simulink model "diskOnPlane_d_V5"  (R2017b)
settings: Solver=VariableStepAuto  StartTime=0.0  StopTime=6  RelTol=1e-3
undefined symbols (not defined in the file): b_contact, cgap, Fz, g, k_contact, mustat, radius, rRim, rTire, s, sigbuilder_block, vthr, X, xPlaLgt, Y, yPlaLgt, Z, zPlaLgt
libraries: sm_lib x23, nesl_utility x14, fl_lib x6, simulink x3, Multibody_Multiphysics_Lib x2, Parts_Lib x1
settings Model: Creator=rizwan  LastModifiedBy=rizwan
settings ExplorerConfigSet: InternalSimMechanicsExplorerSettings="<ExplorerConfiguration><canonicalview>default</canonicalview><AnimationSetting><BasePlaybackSpeed>1.0</BasePlaybackSpeed><PlaybackSpeedFactor>0.5</PlaybackSpeedFactor></AnimationSetting><TilePanel><TileInfo><Tiles Columns=\"1\" Count=\"1\" Rows=\"1\"><Column Weight=\"1\"/><Row Weight=\"1\"/><Tile Height=\"1\" Width=\"1\" X=\"0\" Y=\"0\"/></Tiles></TileInfo><SceneInfo><SceneViewer><BGColor><R>0.60000002384185791</R><G>0.60000002384185791</G><B>0.60000002384185791</B></BGColor><Camera><DoPerspective>off</DoPerspective><Position><X>5.79472373405807684</X><Y>-5.79472391891225325</Y><Z>5.92560694927763798</Z></Position><Center><X>-0.0436274449830504965</X><Y>0.0436272601288755502</Y><Z>0.0872557702365091004</Z></Center><Up><X>-0.408248290463863073</X><Y>0.408248290463863073</Y><Z>0.816496580927726145</Z></Up><ViewLimDist>1</ViewLimDist><YLim>5.77777386756221212</YLim><XLim>8.19359982490539451</XLim></Camera></SceneViewer></SceneInfo></TilePanel><MechEditorPanel><Cameras/><GfxPanelCameraMap/><VideoCreator><PlaybackSpeedRatio>1.0</PlaybackSpeedRatio><FrameRate>30</FrameRate><VideoFormat>Motion JPEG AVI</VideoFormat><FrameSize>auto</FrameSize></VideoCreator></MechEditorPanel></ExplorerConfiguration>"

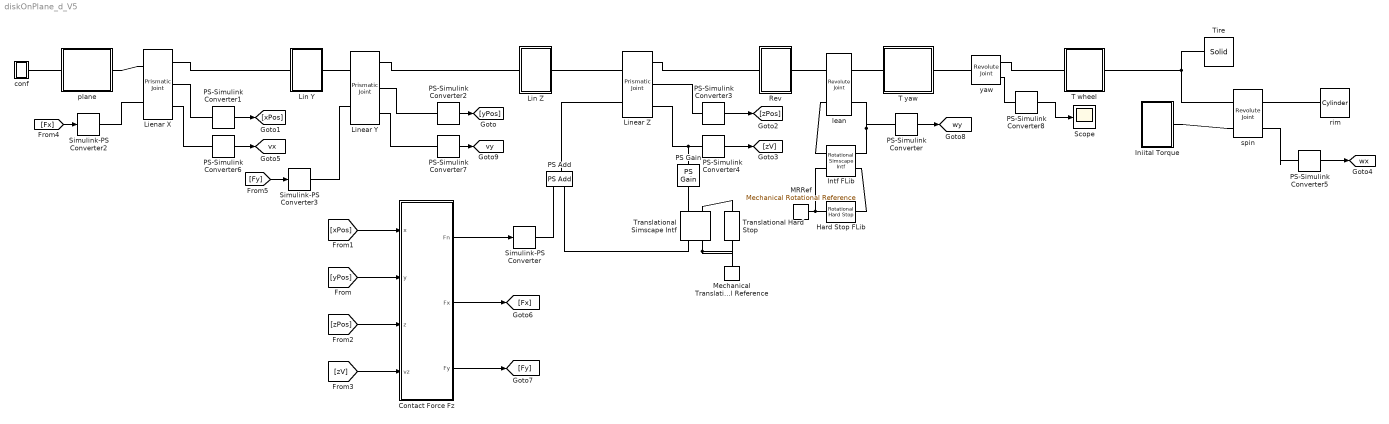
== system diskOnPlane_d_V5 ==
  Contact Force Fz : Subsystem
  Hard Stop FLib : fl_lib/Mechanical/Rotational Elements/Rotational Hard Stop  upper_bnd=70 deg  lower_bnd=-70 deg  stiff_up=1e4 m*N/deg  stiff_low=1e4 m*N/deg  D_up=1e3 m*s*N/deg  D_low=1e3 m*s*N/deg  model=3  transition=0.001 rad  w_specify=off  w_priority=High  w=0 rad/s  w_nominal_specify=off  w_nominal_unit=rad/s  w_nominal_value=1  t_specify=off  t_priority=High  t=0 N*m  t_nominal_specify=off  t_nominal_unit=N*m  t_nominal_value=1  phi_specify=on  phi_priority=High  phi=0 deg  phi_nominal_specify=off  phi_nominal_unit=rad  phi_nominal_value=1
      settings: SourceProductName=Simscape  SourceProductBaseCode=SS
  Iniital Torque : Subsystem
  Intf FLib : Multibody_Multiphysics_Lib/Interfaces/Rotational Simscape Intf  Tag=PublishSubsystem
      settings: SourceProductName=Simscape Multibody Multiphysics Library
  Lienar X : sm_lib/Joints/Prismatic Joint  SenseConstraintForce=off  SenseConstraintForceX=off  SenseConstraintForceY=off  SenseConstraintForceZ=off  SenseConstraintTorque=off  SenseConstraintTorqueX=off  SenseConstraintTorqueY=off  SenseConstraintTorqueZ=off  SenseTotalForce=off  SenseTotalForceX=off  SenseTotalForceY=off  SenseTotalForceZ=off  SenseTotalTorque=off  SenseTotalTorqueX=off  SenseTotalTorqueY=off  SenseTotalTorqueZ=off  CompositeWrenchDir=FollowerOnBase  CompositeWrenchFrame=BaseFrame  EquilibriumPosition=0  EquilibriumPositionUnits=m  SpringStiffness=0  SpringStiffnessUnits=N/m  DampingCoefficient=0  DampingCoefficientUnits=N/(m/s)  TorqueActuationMode=InputTorque  MotionActuationMode=ComputedMotion  SensePosition=on  SenseVelocity=on  SenseAcceleration=off  SenseTorqueForce=off  PositionTargetSpecify=on  PositionTargetPriority=High  PositionTargetValue=sPosX  PositionTargetValueUnits=m  VelocityTargetSpecify=off  VelocityTargetPriority=High  VelocityTargetValue=0  VelocityTargetValueUnits=m/s
  Lin Y : Subsystem
  Lin Z : Subsystem
  Linear Y : sm_lib/Joints/Prismatic Joint  SenseConstraintForce=off  SenseConstraintForceX=off  SenseConstraintForceY=off  SenseConstraintForceZ=off  SenseConstraintTorque=off  SenseConstraintTorqueX=off  SenseConstraintTorqueY=off  SenseConstraintTorqueZ=off  SenseTotalForce=off  SenseTotalForceX=off  SenseTotalForceY=off  SenseTotalForceZ=off  SenseTotalTorque=off  SenseTotalTorqueX=off  SenseTotalTorqueY=off  SenseTotalTorqueZ=off  CompositeWrenchDir=FollowerOnBase  CompositeWrenchFrame=BaseFrame  EquilibriumPosition=0  EquilibriumPositionUnits=m  SpringStiffness=0  SpringStiffnessUnits=N/m  DampingCoefficient=0  DampingCoefficientUnits=N/(m/s)  TorqueActuationMode=InputTorque  MotionActuationMode=ComputedMotion  SensePosition=on  SenseVelocity=on  SenseAcceleration=off  SenseTorqueForce=off  PositionTargetSpecify=off  PositionTargetPriority=High  PositionTargetValue=0  PositionTargetValueUnits=m  VelocityTargetSpecify=off  VelocityTargetPriority=High  VelocityTargetValue=0  VelocityTargetValueUnits=m/s
  Linear Z : sm_lib/Joints/Prismatic Joint  SenseConstraintForce=off  SenseConstraintForceX=off  SenseConstraintForceY=off  SenseConstraintForceZ=off  SenseConstraintTorque=off  SenseConstraintTorqueX=off  SenseConstraintTorqueY=off  SenseConstraintTorqueZ=off  SenseTotalForce=off  SenseTotalForceX=off  SenseTotalForceY=off  SenseTotalForceZ=off  SenseTotalTorque=off  SenseTotalTorqueX=off  SenseTotalTorqueY=off  SenseTotalTorqueZ=off  CompositeWrenchDir=FollowerOnBase  CompositeWrenchFrame=BaseFrame  EquilibriumPosition=0  EquilibriumPositionUnits=m  SpringStiffness=0  SpringStiffnessUnits=N/m  DampingCoefficient=0  DampingCoefficientUnits=N/(m/s)  TorqueActuationMode=InputTorque  MotionActuationMode=ComputedMotion  SensePosition=on  SenseVelocity=on  SenseAcceleration=off  SenseTorqueForce=off  PositionTargetSpecify=off  PositionTargetPriority=High  PositionTargetValue=0  PositionTargetValueUnits=m  VelocityTargetSpecify=off  VelocityTargetPriority=High  VelocityTargetValue=0  VelocityTargetValueUnits=m/s
  MRRef : fl_lib/Mechanical/Rotational Elements/Mechanical Rotational Reference
  Mechanical Translational Reference : fl_lib/Mechanical/Translational Elements/Mechanical Translational Reference
  PS Add : fl_lib/Physical Signals/Functions/PS Add
  PS Gain : fl_lib/Physical Signals/Functions/PS Gain  gain=1
  PS-Simulink Converter{,1..7} (8 alike) : nesl_utility/PS-Simulink Converter  PhysicalDomain=network_engine_domain  SubClassName=ps_output  LeftPortType=input  RightPortType=output  PseudoPeriodic=off  Frequencies=[]  Unit=1  AffineConversion=off
  PS-Simulink Converter8 : nesl_utility/PS-Simulink Converter  PhysicalDomain=network_engine_domain  SubClassName=ps_output  LeftPortType=input  RightPortType=output  PseudoPeriodic=off  Frequencies=[]  Unit=deg  AffineConversion=off
  Rev : Subsystem
  Scope : Scope
  Simulink-PS Converter : nesl_utility/Simulink-PS Converter  PhysicalDomain=network_engine_domain  SubClassName=ps_input  LeftPortType=input  RightPortType=output  PseudoPeriodic=off  Frequencies=[]  NoiseDistribution=none  NoiseParameters=[]  Unit=1  AffineConversion=off  FilteringAndDerivatives=provide  SimscapeFilterOrder=1  InputFilterTimeConstant=0.001  UdotUserProvided=0
  Simulink-PS Converter2 : nesl_utility/Simulink-PS Converter  PhysicalDomain=network_engine_domain  SubClassName=ps_input  LeftPortType=input  RightPortType=output  PseudoPeriodic=off  Frequencies=[]  NoiseDistribution=none  NoiseParameters=[]  Unit=1  AffineConversion=off  FilteringAndDerivatives=provide  SimscapeFilterOrder=1  InputFilterTimeConstant=0.001  UdotUserProvided=0
  Simulink-PS Converter3 : nesl_utility/Simulink-PS Converter  PhysicalDomain=network_engine_domain  SubClassName=ps_input  LeftPortType=input  RightPortType=output  PseudoPeriodic=off  Frequencies=[]  NoiseDistribution=none  NoiseParameters=[]  Unit=1  AffineConversion=off  FilteringAndDerivatives=provide  SimscapeFilterOrder=1  InputFilterTimeConstant=0.001  UdotUserProvided=0
  T wheel : Subsystem
  T yaw : Subsystem
  Tire : sm_lib/Body Elements/Solid  InertiaType=CalculateFromGeometry  Mass=1  MassUnits=kg  CenterOfMass=[0 0 0]  CenterOfMassUnits=m  MomentsOfInertia=[1 1 1]  MomentsOfInertiaUnits=kg*m^2  ProductsOfInertia=[1 1 1]  ProductsOfInertiaUnits=kg*m^2  DensityBased=on  Density=rhoTire  DensityUnits=kg/m^3  DoExposeReferenceFrame=on  SerializedFrames=<Frames/>  GraphicType=FromGeometry  MarkerShape=Sphere  MarkerSize=10  GraphicVisPropType=SimpleVisualProperties  GraphicDiffuseColor=[1.0 0.2 0.2]  GraphicSpecularColor=[0.5 0.5 0.5 1.0]  GraphicAmbientColor=[0.15 0.15 0.15 1.0]  GraphicEmissiveColor=[0.0 0.0 0.0 1.0]  GraphicShininess=75  GraphicOpacity=0.3  GeometryShape=GeneralSolidOfRevolution  RectangleSize=[1 1]  RectangleSizeUnits=m  BrickDimensions=[1 1 1]  BrickDimensionUnits=m  CylinderRadius=1  CylinderRadiusUnits=m  CylinderLength=1  CylinderLengthUnits=m  SphereRadius=1  SphereRadiusUnits=m  EllipsoidRadii=[1 1 1]  EllipsoidRadiiUnits=m  ExtrusionCrossSection=[1 1; -1 1; -1 -1; 1 -1]  ExtrusionCrossSectionUnits=m  ExtrusionLength=1  ExtrusionLengthUnits=m  PolygonNumSides=3  PolygonOuterRadius=1  PolygonOuterRadiusUnits=m  ExtGeomFileType=STEP  ExtGeomFileUnits=m  RevolutionCrossSection=aTire  RevolutionCrossSectionUnits=m  RevolutionExtent=Full  RevolutionAngle=180  RevolutionAngleUnits=deg
  Translational Simscape Intf : Multibody_Multiphysics_Lib/Interfaces/Translational Simscape Intf
  Translational Hard Stop : fl_lib/Mechanical/Translational Elements/Translational Hard Stop  upper_bnd=+inf m  lower_bnd=-inf cm  stiff_up=1e6 N/m  stiff_low=1e6 N/m  D_up=150 N/(m/s)  D_low=150 N/(m/s)  model=3  transition=0.1 mm  v_specify=off  v_priority=None  v=0 m/s  v_nominal_specify=off  v_nominal_unit=m/s  v_nominal_value=1  f_specify=off  f_priority=None  f=0 N  f_nominal_specify=off  f_nominal_unit=N  f_nominal_value=1  x_specify=off  x_priority=High  x=0 m  x_nominal_specify=off  x_nominal_unit=m  x_nominal_value=1
  conf : Subsystem
  lean : sm_lib/Joints/Revolute Joint  SenseConstraintForce=off  SenseConstraintForceX=off  SenseConstraintForceY=off  SenseConstraintForceZ=off  SenseConstraintTorque=off  SenseConstraintTorqueX=off  SenseConstraintTorqueY=off  SenseConstraintTorqueZ=off  SenseTotalForce=off  SenseTotalForceX=off  SenseTotalForceY=off  SenseTotalForceZ=off  SenseTotalTorque=off  SenseTotalTorqueX=off  SenseTotalTorqueY=off  SenseTotalTorqueZ=off  CompositeWrenchDir=FollowerOnBase  CompositeWrenchFrame=BaseFrame  EquilibriumPosition=0  EquilibriumPositionUnits=deg  SpringStiffness=0  SpringStiffnessUnits=N*m/deg  DampingCoefficient=0  DampingCoefficientUnits=N*m/(deg/s)  TorqueActuationMode=InputTorque  MotionActuationMode=ComputedMotion  SensePosition=off  SenseVelocity=on  SenseAcceleration=off  SenseTorqueForce=off  PositionTargetSpecify=on  PositionTargetPriority=High  PositionTargetValue=dAngle  PositionTargetValueUnits=deg  VelocityTargetSpecify=off  VelocityTargetPriority=High  VelocityTargetValue=0  VelocityTargetValueUnits=deg/s
  plane : Subsystem
  rim : Parts_Lib/Cylinder  Tag=CustomStyle  cyl_radius=rRim  cyl_length=lRim  cyl_density=rhoDisk  cyl_color=blue  cyl_opacity=1  cyl_color_custom="[0.7920    0.9900    0.9900]"  mark_radius=[0.75 0.5]  mark_len_factor=1.01  mark_angle=60  mark_color=purple  mark_opacity=1
  spin : sm_lib/Joints/Revolute Joint  SenseConstraintForce=off  SenseConstraintForceX=off  SenseConstraintForceY=off  SenseConstraintForceZ=off  SenseConstraintTorque=off  SenseConstraintTorqueX=off  SenseConstraintTorqueY=off  SenseConstraintTorqueZ=off  SenseTotalForce=off  SenseTotalForceX=off  SenseTotalForceY=off  SenseTotalForceZ=off  SenseTotalTorque=off  SenseTotalTorqueX=off  SenseTotalTorqueY=off  SenseTotalTorqueZ=off  CompositeWrenchDir=FollowerOnBase  CompositeWrenchFrame=BaseFrame  EquilibriumPosition=0  EquilibriumPositionUnits=deg  SpringStiffness=0  SpringStiffnessUnits=N*m/deg  DampingCoefficient=0  DampingCoefficientUnits=N*m/(deg/s)  TorqueActuationMode=InputTorque  MotionActuationMode=ComputedMotion  SensePosition=off  SenseVelocity=on  SenseAcceleration=off  SenseTorqueForce=off  PositionTargetSpecify=off  PositionTargetPriority=High  PositionTargetValue=0  PositionTargetValueUnits=deg  VelocityTargetSpecify=off  VelocityTargetPriority=High  VelocityTargetValue=0  VelocityTargetValueUnits=deg/s
  yaw : sm_lib/Joints/Revolute Joint  SenseConstraintForce=off  SenseConstraintForceX=off  SenseConstraintForceY=off  SenseConstraintForceZ=off  SenseConstraintTorque=off  SenseConstraintTorqueX=off  SenseConstraintTorqueY=off  SenseConstraintTorqueZ=off  SenseTotalForce=off  SenseTotalForceX=off  SenseTotalForceY=off  SenseTotalForceZ=off  SenseTotalTorque=off  SenseTotalTorqueX=off  SenseTotalTorqueY=off  SenseTotalTorqueZ=off  CompositeWrenchDir=FollowerOnBase  CompositeWrenchFrame=BaseFrame  EquilibriumPosition=0  EquilibriumPositionUnits=deg  SpringStiffness=0  SpringStiffnessUnits=N*m/deg  DampingCoefficient=0  DampingCoefficientUnits=N*m/(deg/s)  TorqueActuationMode=NoTorque  MotionActuationMode=ComputedMotion  SensePosition=on  SenseVelocity=off  SenseAcceleration=off  SenseTorqueForce=off  PositionTargetSpecify=off  PositionTargetPriority=High  PositionTargetValue=0  PositionTargetValueUnits=deg  VelocityTargetSpecify=off  VelocityTargetPriority=High  VelocityTargetValue=0  VelocityTargetValueUnits=deg/s
  tag scope: vx=global, vy=global, wx=global, wy=global
  wires:
  PS-Simulink Converter5/1 -> [wx]
  PS-Simulink Converter/1 -> [wy]
  [Fx] -> Simulink-PS Converter2/1
  PS-Simulink Converter1/1 -> [xPos]
  PS-Simulink Converter6/1 -> [vx]
  [Fy] -> Simulink-PS Converter3/1
  PS-Simulink Converter2/1 -> [yPos]
  PS-Simulink Converter7/1 -> [vy]
  PS-Simulink Converter4/1 -> [zV]
  PS-Simulink Converter3/1 -> [zPos]
  Contact Force Fz/1(Fn) -> Simulink-PS Converter/1
  [xPos] -> Contact Force Fz/1(x)
  [yPos] -> Contact Force Fz/2(y)
  Contact Force Fz/3(Fy) -> [Fy]
  [zV] -> Contact Force Fz/4(vz)
  [zPos] -> Contact Force Fz/3(z)
  Contact Force Fz/2(Fx) -> [Fx]
  PS-Simulink Converter8/1 -> Scope/1
  connections:
  Tire/RConn1 -- T wheel/RConn1 -- spin/LConn1
  plane/LConn1 -- conf/RConn1
  plane/RConn1 -- Lienar X/LConn1
  Lienar X/RConn1 -- Lin Y/LConn1
  Linear Y/LConn1 -- Lin Y/RConn1
  Lin Z/LConn1 -- Linear Y/RConn1
  Linear Z/LConn1 -- Lin Z/RConn1
  Rev/LConn1 -- Linear Z/RConn1
  lean/LConn1 -- Rev/RConn1
  T yaw/LConn1 -- lean/RConn1
  T yaw/RConn1 -- yaw/LConn1
  spin/RConn1 -- rim/LConn1
  spin/RConn2 -- PS-Simulink Converter5/LConn1
  yaw/RConn1 -- T wheel/LConn1
  lean/RConn2 -- PS-Simulink Converter/LConn1 -- Intf FLib/RConn1
  Intf FLib/LConn1 -- lean/LConn2
  Hard Stop FLib/LConn1 -- Intf FLib/RConn2
  Hard Stop FLib/RConn1 -- MRRef/LConn1 -- Intf FLib/LConn2
  Simulink-PS Converter2/RConn1 -- Lienar X/LConn2
  Lienar X/RConn2 -- PS-Simulink Converter1/LConn1
  Lienar X/RConn3 -- PS-Simulink Converter6/LConn1
  Iniital Torque/RConn1 -- spin/LConn2
  Linear Y/LConn2 -- Simulink-PS Converter3/RConn1
  Linear Y/RConn2 -- PS-Simulink Converter2/LConn1
  PS-Simulink Converter7/LConn1 -- Linear Y/RConn3
  Linear Z/RConn2 -- PS-Simulink Converter3/LConn1
  Linear Z/RConn3 -- PS Gain/LConn1 -- PS-Simulink Converter4/LConn1
  Translational Simscape Intf/LConn2 -- Translational Hard Stop/RConn1 -- Mechanical Translational Reference/LConn1
  PS Gain/RConn1 -- Translational Simscape Intf/RConn1
  Translational Simscape Intf/LConn1 -- PS Add/LConn1
  Translational Hard Stop/LConn1 -- Translational Simscape Intf/RConn2
  Simulink-PS Converter/RConn1 -- PS Add/LConn2
  PS Add/RConn1 -- Linear Z/LConn2
  PS-Simulink Converter8/LConn1 -- yaw/RConn2

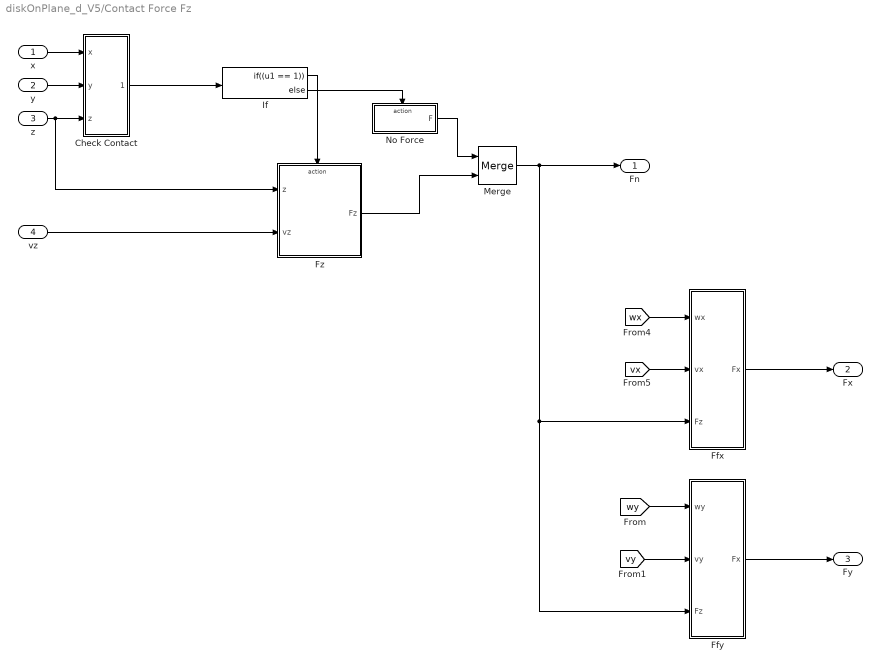
== system diskOnPlane_d_V5/Contact Force Fz ==
  x : Inport
  y : Inport  Port=2
  z : Inport  Port=3
  vz : Inport  Port=4
  Check Contact : Subsystem
  Ffx : Subsystem
  Ffy : Subsystem
  Fz : Subsystem
  If : If  IfExpression=(u1 == 1)
  Merge : Merge  InitialOutput=0  InputPortOffsets=0
  No Force : Subsystem  AncestorBlock=Contact_Forces_Lib/2D/Circle to Finite Line Force/No Force
  Fn : Outport
  Fx : Outport  Port=2
  Fy : Outport  Port=3
  wires:
  Fz/1(Fz) -> Merge/2
  If/1 -> Fz/Action
  Check Contact/1(Enable) -> If/1
  No Force/1(F) -> Merge/1
  Merge/1 -> Ffy/3(Fz), Ffx/3(Fz), Fn/1
  x/1 -> Check Contact/1(x)
  If/2 -> No Force/Action
  y/1 -> Check Contact/2(y)
  z/1 -> Fz/1(z), Check Contact/3(z)
  vz/1 -> Fz/2(vz)
  [vx] -> Ffx/2(vx)
  [wx] -> Ffx/1(wx)
  Ffx/1(Fx) -> Fx/1
  [wy] -> Ffy/1(wy)
  [vy] -> Ffy/2(vy)
  Ffy/1(Fx) -> Fy/1

== system diskOnPlane_d_V5/Iniital Torque ==
  Gain : Gain  Gain=1/2.5
  Signal Builder : Subsystem  Tag=STV Subsys  LoadFcn=sigbuilder_block('load');  StartFcn=sigbuilder_block('start');  StopFcn=sigbuilder_block('stop');  ClipboardFcn=sigbuilder_block('clipboard');  mask(Sigbuilder block){tuvar=[0:10]}
      mask help: Simulink:masks:SigbuilderBlock_MD
      mask init:
      | if ~strcmp(get_param(bdroot(gcbh),'SimulationStatus'),'stopped') tuvar = sigbuilder_block('maskInit'); end
      settings: CopyFcn=sigbuilder_block('copy');  DeleteFcn=sigbuilder_block('delete');  ModelCloseFcn=sigbuilder_block('modelClose');  PreSaveFcn=sigbuilder_block('preSave');  PauseFcn=sigbuilder_block('pause');  ContinueFcn=sigbuilder_block('continue');  NameChangeFcn=sigbuilder_block('namechange');  OpenFcn=sigbuilder_block('open',[48.75 0 975.75 495.75 ]);  CloseFcn=sigbuilder_block('close');
      mask Display: plot(0, 0, 100, 100,[2, 2, 32, 32, 2], [68, 8, 8, 68, 68],[32, 2], [38, 38], [32, 19, 2],[53, 60, 44], [32, 17, 17, 2],[16, 16, 31, 31]);txt = getActiveGroup(gcbh);text(2, 100, txt,'verticalAlignment', 'top');
  Simulink-PS Converter1 : nesl_utility/Simulink-PS Converter  PhysicalDomain=network_engine_domain  SubClassName=ps_input  LeftPortType=input  RightPortType=output  PseudoPeriodic=off  Frequencies=[]  NoiseDistribution=none  NoiseParameters=[]  Unit=N*m  AffineConversion=off  FilteringAndDerivatives=filter  SimscapeFilterOrder=2  InputFilterTimeConstant=0.1  UdotUserProvided=0
  wheel : PMIOPort  Port=1  Side=Right
  wires:
  Gain/1 -> Simulink-PS Converter1/1
  Signal Builder/1(Signal 1) -> Gain/1
  connections:
  Simulink-PS Converter1/RConn1 -- wheel/RConn1

== system diskOnPlane_d_V5/Lin Y ==
  Rev for Linear X : sm_lib/Frames and Transforms/Rigid Transform  TranslationMethod=None  TranslationStandardOffset=0  TranslationLengthUnit=m  TranslationStandardAxis=+Z  TranslationCartesianOffset=[0 0 0]  TranslationROffset=0  TranslationROffsetUnits=m  TranslationZOffset=0  TranslationZOffsetUnits=m  TranslationThetaOffset=0  TranslationThetaOffsetUnits=deg  RotationMethod=StandardAxis  RotationAngleUnits=deg  RotationStandardAxis=-Y  RotationAngle=90  RotationArbitraryAxis=[0 0 1]  FollAlignAxisA=+X  BaseAlignAxisA=+Y  FollAlignAxisB=+Y  BaseAlignAxisB=+Z  RotationSequenceAxes=FollowerAxes  RotationSequence=XYX  RotationSequenceAngles=[0 0 0]  RotationSequenceAnglesUnits=deg  RotationMatrix=[1 0 0; 0 1 0; 0 0 1]
  Trans for Linear Y : sm_lib/Frames and Transforms/Rigid Transform  TranslationMethod=StandardAxis  TranslationStandardOffset=rTire  TranslationLengthUnit=m  TranslationStandardAxis=-Y  TranslationCartesianOffset=[0 0 0]  TranslationROffset=0  TranslationROffsetUnits=m  TranslationZOffset=0  TranslationZOffsetUnits=m  TranslationThetaOffset=0  TranslationThetaOffsetUnits=deg  RotationMethod=None  RotationAngleUnits=deg  RotationStandardAxis=+Z  RotationAngle=0.0  RotationArbitraryAxis=[0 0 1]  FollAlignAxisA=+X  BaseAlignAxisA=+Y  FollAlignAxisB=+Y  BaseAlignAxisB=+Z  RotationSequenceAxes=FollowerAxes  RotationSequence=XYX  RotationSequenceAngles=[0 0 0]  RotationSequenceAnglesUnits=deg  RotationMatrix=[1 0 0; 0 1 0; 0 0 1]
  B : PMIOPort  Port=1  Side=Left
  F : PMIOPort  Port=2  Side=Right
  connections:
  B/RConn1 -- Rev for Linear X/LConn1
  F/RConn1 -- Trans for Linear Y/RConn1
  Trans for Linear Y/LConn1 -- Rev for Linear X/RConn1

== system diskOnPlane_d_V5/Lin Z ==
  Rev for Linear Y : sm_lib/Frames and Transforms/Rigid Transform  TranslationMethod=StandardAxis  TranslationStandardOffset=rTire  TranslationLengthUnit=m  TranslationStandardAxis=+Y  TranslationCartesianOffset=[0 0 0]  TranslationROffset=0  TranslationROffsetUnits=m  TranslationZOffset=0  TranslationZOffsetUnits=m  TranslationThetaOffset=0  TranslationThetaOffsetUnits=deg  RotationMethod=None  RotationAngleUnits=deg  RotationStandardAxis=+Z  RotationAngle=0.0  RotationArbitraryAxis=[0 0 1]  FollAlignAxisA=+X  BaseAlignAxisA=+Y  FollAlignAxisB=+Y  BaseAlignAxisB=+Z  RotationSequenceAxes=FollowerAxes  RotationSequence=XYX  RotationSequenceAngles=[0 0 0]  RotationSequenceAnglesUnits=deg  RotationMatrix=[1 0 0; 0 1 0; 0 0 1]
  Trans for Lineaer Z : sm_lib/Frames and Transforms/Rigid Transform  TranslationMethod=None  TranslationStandardOffset=0  TranslationLengthUnit=m  TranslationStandardAxis=+Z  TranslationCartesianOffset=[0 0 0]  TranslationROffset=0  TranslationROffsetUnits=m  TranslationZOffset=0  TranslationZOffsetUnits=m  TranslationThetaOffset=0  TranslationThetaOffsetUnits=deg  RotationMethod=StandardAxis  RotationAngleUnits=deg  RotationStandardAxis=-X  RotationAngle=90  RotationArbitraryAxis=[0 0 1]  FollAlignAxisA=+X  BaseAlignAxisA=+Y  FollAlignAxisB=+Y  BaseAlignAxisB=+Z  RotationSequenceAxes=FollowerAxes  RotationSequence=XYX  RotationSequenceAngles=[0 0 0]  RotationSequenceAnglesUnits=deg  RotationMatrix=[1 0 0; 0 1 0; 0 0 1]
  B : PMIOPort  Port=1  Side=Left
  F : PMIOPort  Port=2  Side=Right
  connections:
  Rev for Linear Y/LConn1 -- B/RConn1
  F/RConn1 -- Trans for Lineaer Z/RConn1
  Trans for Lineaer Z/LConn1 -- Rev for Linear Y/RConn1

== system diskOnPlane_d_V5/Rev ==
  Rev for Linear Z : sm_lib/Frames and Transforms/Rigid Transform  TranslationMethod=None  TranslationStandardOffset=0  TranslationLengthUnit=m  TranslationStandardAxis=+Z  TranslationCartesianOffset=[0 0 0]  TranslationROffset=0  TranslationROffsetUnits=m  TranslationZOffset=0  TranslationZOffsetUnits=m  TranslationThetaOffset=0  TranslationThetaOffsetUnits=deg  RotationMethod=StandardAxis  RotationAngleUnits=deg  RotationStandardAxis=+X  RotationAngle=90  RotationArbitraryAxis=[0 0 1]  FollAlignAxisA=+X  BaseAlignAxisA=+Y  FollAlignAxisB=+Y  BaseAlignAxisB=+Z  RotationSequenceAxes=FollowerAxes  RotationSequence=XYX  RotationSequenceAngles=[0 0 0]  RotationSequenceAnglesUnits=deg  RotationMatrix=[1 0 0; 0 1 0; 0 0 1]
  Trans for lean axis : sm_lib/Frames and Transforms/Rigid Transform  TranslationMethod=StandardAxis  TranslationStandardOffset=rTire  TranslationLengthUnit=m  TranslationStandardAxis=-Y  TranslationCartesianOffset=[0 0 0]  TranslationROffset=0  TranslationROffsetUnits=m  TranslationZOffset=0  TranslationZOffsetUnits=m  TranslationThetaOffset=0  TranslationThetaOffsetUnits=deg  RotationMethod=StandardAxis  RotationAngleUnits=deg  RotationStandardAxis=+Y  RotationAngle=90  RotationArbitraryAxis=[0 0 1]  FollAlignAxisA=+X  BaseAlignAxisA=+Y  FollAlignAxisB=+Y  BaseAlignAxisB=+Z  RotationSequenceAxes=FollowerAxes  RotationSequence=XYX  RotationSequenceAngles=[0 0 0]  RotationSequenceAnglesUnits=deg  RotationMatrix=[1 0 0; 0 1 0; 0 0 1]
  B : PMIOPort  Port=1  Side=Left
  F : PMIOPort  Port=2  Side=Right
  connections:
  Trans for lean axis/LConn1 -- Rev for Linear Z/RConn1
  F/RConn1 -- Trans for lean axis/RConn1
  Rev for Linear Z/LConn1 -- B/RConn1

== system diskOnPlane_d_V5/T wheel ==
  RTrans for yaw axis : sm_lib/Frames and Transforms/Rigid Transform  TranslationMethod=StandardAxis  TranslationStandardOffset=rTire  TranslationLengthUnit=m  TranslationStandardAxis=+Y  TranslationCartesianOffset=[0 0 0]  TranslationROffset=0  TranslationROffsetUnits=m  TranslationZOffset=0  TranslationZOffsetUnits=m  TranslationThetaOffset=0  TranslationThetaOffsetUnits=deg  RotationMethod=None  RotationAngleUnits=deg  RotationStandardAxis=+Z  RotationAngle=0.0  RotationArbitraryAxis=[0 0 1]  FollAlignAxisA=+X  BaseAlignAxisA=+Y  FollAlignAxisB=+Y  BaseAlignAxisB=+Z  RotationSequenceAxes=FollowerAxes  RotationSequence=XYX  RotationSequenceAngles=[0 0 0]  RotationSequenceAnglesUnits=deg  RotationMatrix=[1 0 0; 0 1 0; 0 0 1]
  Rot for yaw axis1 : sm_lib/Frames and Transforms/Rigid Transform  TranslationMethod=None  TranslationStandardOffset=0  TranslationLengthUnit=m  TranslationStandardAxis=+Z  TranslationCartesianOffset=[0 0 0]  TranslationROffset=0  TranslationROffsetUnits=m  TranslationZOffset=0  TranslationZOffsetUnits=m  TranslationThetaOffset=0  TranslationThetaOffsetUnits=deg  RotationMethod=StandardAxis  RotationAngleUnits=deg  RotationStandardAxis=+X  RotationAngle=90  RotationArbitraryAxis=[0 0 1]  FollAlignAxisA=+X  BaseAlignAxisA=+Y  FollAlignAxisB=+Y  BaseAlignAxisB=+Z  RotationSequenceAxes=FollowerAxes  RotationSequence=XYX  RotationSequenceAngles=[0 0 0]  RotationSequenceAnglesUnits=deg  RotationMatrix=[1 0 0; 0 1 0; 0 0 1]
  B : PMIOPort  Port=1  Side=Left
  F : PMIOPort  Port=2  Side=Right
  connections:
  B/RConn1 -- Rot for yaw axis1/LConn1
  Rot for yaw axis1/RConn1 -- RTrans for yaw axis/LConn1
  RTrans for yaw axis/RConn1 -- F/RConn1

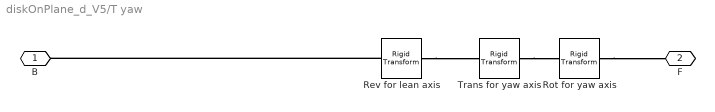
== system diskOnPlane_d_V5/T yaw ==
  Rev for lean axis : sm_lib/Frames and Transforms/Rigid Transform  TranslationMethod=StandardAxis  TranslationStandardOffset=rTire  TranslationLengthUnit=m  TranslationStandardAxis=+Y  TranslationCartesianOffset=[0 0 0]  TranslationROffset=0  TranslationROffsetUnits=m  TranslationZOffset=0  TranslationZOffsetUnits=m  TranslationThetaOffset=0  TranslationThetaOffsetUnits=deg  RotationMethod=StandardAxis  RotationAngleUnits=deg  RotationStandardAxis=-Y  RotationAngle=90  RotationArbitraryAxis=[0 0 1]  FollAlignAxisA=+X  BaseAlignAxisA=+Y  FollAlignAxisB=+Y  BaseAlignAxisB=+Z  RotationSequenceAxes=FollowerAxes  RotationSequence=XYX  RotationSequenceAngles=[0 0 0]  RotationSequenceAnglesUnits=deg  RotationMatrix=[1 0 0; 0 1 0; 0 0 1]
  Rot for yaw axis : sm_lib/Frames and Transforms/Rigid Transform  TranslationMethod=None  TranslationStandardOffset=0  TranslationLengthUnit=m  TranslationStandardAxis=+Z  TranslationCartesianOffset=[0 0 0]  TranslationROffset=0  TranslationROffsetUnits=m  TranslationZOffset=0  TranslationZOffsetUnits=m  TranslationThetaOffset=0  TranslationThetaOffsetUnits=deg  RotationMethod=StandardAxis  RotationAngleUnits=deg  RotationStandardAxis=-X  RotationAngle=90  RotationArbitraryAxis=[0 0 1]  FollAlignAxisA=+X  BaseAlignAxisA=+Y  FollAlignAxisB=+Y  BaseAlignAxisB=+Z  RotationSequenceAxes=FollowerAxes  RotationSequence=XYX  RotationSequenceAngles=[0 0 0]  RotationSequenceAnglesUnits=deg  RotationMatrix=[1 0 0; 0 1 0; 0 0 1]
  Trans for yaw axis : sm_lib/Frames and Transforms/Rigid Transform  TranslationMethod=StandardAxis  TranslationStandardOffset=rTire  TranslationLengthUnit=m  TranslationStandardAxis=-Y  TranslationCartesianOffset=[0 0 0]  TranslationROffset=0  TranslationROffsetUnits=m  TranslationZOffset=0  TranslationZOffsetUnits=m  TranslationThetaOffset=0  TranslationThetaOffsetUnits=deg  RotationMethod=None  RotationAngleUnits=deg  RotationStandardAxis=+Z  RotationAngle=0.0  RotationArbitraryAxis=[0 0 1]  FollAlignAxisA=+X  BaseAlignAxisA=+Y  FollAlignAxisB=+Y  BaseAlignAxisB=+Z  RotationSequenceAxes=FollowerAxes  RotationSequence=XYX  RotationSequenceAngles=[0 0 0]  RotationSequenceAnglesUnits=deg  RotationMatrix=[1 0 0; 0 1 0; 0 0 1]
  B : PMIOPort  Port=1  Side=Left
  F : PMIOPort  Port=2  Side=Right
  connections:
  Trans for yaw axis/RConn1 -- Rot for yaw axis/LConn1
  Rot for yaw axis/RConn1 -- F/RConn1
  Rev for lean axis/LConn1 -- B/RConn1
  Rev for lean axis/RConn1 -- Trans for yaw axis/LConn1

== system diskOnPlane_d_V5/conf ==
  Mechanism Configuration : sm_lib/Utilities/Mechanism Configuration  UniformGravity=Constant  GravityVector=[0 0 -g]  GravityUnits=m/s^2  LinearizationDelta=0.001
  Solver Configuration : nesl_utility/Solver Configuration  PhysicalDomain=network_engine_domain  SubClassName=solver  LeftPortType=input  RightPortType=generic  Accelerate=off  Tones=[]  Harmonics=[]  SimulateNoise=off  Profile=off  UseLocalSampling=off  EnableSwitchedLinearOptims=on  FrequencyDomain=off  UseCCode=off  RelTol=0.001  AbsTol=1e-06  MinStep=1e-09  ToWorkspace=off  RevertToSquareIcSolve=off  NumHomotopyIterations=100  PhasorMode=off  PhasorModeNumHarmonics=1  DoDC=off  ResidualTolerance=1e-9  UseLocalSolver=off  LocalSolverChoice=NE_BACKWARD_EULER_ADVANCER  LocalSolverSampleTime=.001  DoFixedCost=off  MaxNonlinIter=3  MaxModeIter=2  LinearAlgebra=Sparse  DelaysMemoryBudget=1024  AutomaticFiltering=on  FilteringTimeConstant=0.001
  World Frame : sm_lib/Frames and Transforms/World Frame
  c : PMIOPort  Port=1  Side=Right
  connections:
  Mechanism Configuration/RConn1 -- Solver Configuration/RConn1 -- c/RConn1 -- World Frame/RConn1

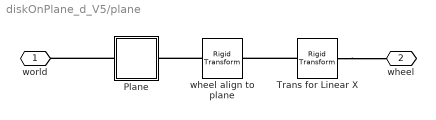
== system diskOnPlane_d_V5/plane ==
  Plane : Subsystem
  Trans for Linear X : sm_lib/Frames and Transforms/Rigid Transform  TranslationMethod=None  TranslationStandardOffset=0  TranslationLengthUnit=m  TranslationStandardAxis=+Z  TranslationCartesianOffset=[0 0 0]  TranslationROffset=0  TranslationROffsetUnits=m  TranslationZOffset=0  TranslationZOffsetUnits=m  TranslationThetaOffset=0  TranslationThetaOffsetUnits=deg  RotationMethod=StandardAxis  RotationAngleUnits=deg  RotationStandardAxis=+Y  RotationAngle=90  RotationArbitraryAxis=[0 0 1]  FollAlignAxisA=+X  BaseAlignAxisA=+Y  FollAlignAxisB=+Y  BaseAlignAxisB=+Z  RotationSequenceAxes=FollowerAxes  RotationSequence=XYX  RotationSequenceAngles=[0 0 0]  RotationSequenceAnglesUnits=deg  RotationMatrix=[1 0 0; 0 1 0; 0 0 1]
  wheel align to plane : sm_lib/Frames and Transforms/Rigid Transform  TranslationMethod=Cartesian  TranslationStandardOffset=radius+zPlaLgt/2  TranslationLengthUnit=m  TranslationStandardAxis=+Z  TranslationCartesianOffset=[0 0 rRim+s+zPlaLgt/2]  TranslationROffset=0  TranslationROffsetUnits=m  TranslationZOffset=0  TranslationZOffsetUnits=m  TranslationThetaOffset=0  TranslationThetaOffsetUnits=deg  RotationMethod=StandardAxis  RotationAngleUnits=deg  RotationStandardAxis=+X  RotationAngle=90  RotationArbitraryAxis=[0 0 1]  FollAlignAxisA=+X  BaseAlignAxisA=+Y  FollAlignAxisB=+Y  BaseAlignAxisB=+Z  RotationSequenceAxes=FollowerAxes  RotationSequence=XYX  RotationSequenceAngles=[0 0 0]  RotationSequenceAnglesUnits=deg  RotationMatrix=[1 0 0; 0 1 0; 0 0 1]
  world : PMIOPort  Port=1  Side=Left
  wheel : PMIOPort  Port=2  Side=Right
  connections:
  Plane/LConn1 -- world/RConn1
  wheel align to plane/LConn1 -- Plane/RConn1
  Trans for Linear X/LConn1 -- wheel align to plane/RConn1
  Trans for Linear X/RConn1 -- wheel/RConn1

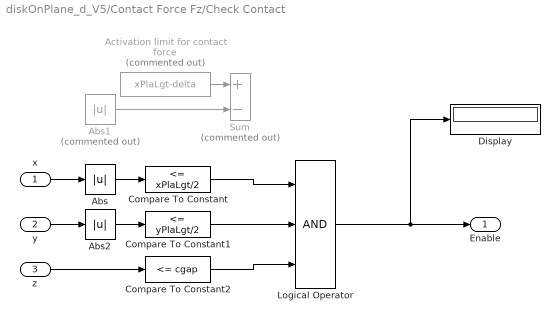
== system diskOnPlane_d_V5/Contact Force Fz/Check Contact ==
  x : Inport
  y : Inport  Port=2
  z : Inport  Port=3
  Abs : Abs
  Abs1 : Abs  Commented=on  ZeroCross=off
  Abs2 : Abs
  Activation limit for contact force : Constant  Commented=on  Value=xPlaLgt-delta
  Compare To Constant : simulink/Logic and Bit Operations/Compare To Constant  relop=<=  const=xPlaLgt/2  OutDataTypeStr=boolean
  Compare To Constant1 : simulink/Logic and Bit Operations/Compare To Constant  relop=<=  const=yPlaLgt/2  OutDataTypeStr=boolean
  Compare To Constant2 : simulink/Logic and Bit Operations/Compare To Constant  relop=<=  const=cgap  OutDataTypeStr=boolean
  Display : Display
  Logical Operator : Logic  Inputs=3  AllPortsSameDT=off  OutDataTypeStr=boolean
  Sum : Sum  Commented=on  Inputs=+-
  Enable : Outport
  wires:
  Activation limit for contact force/1 -> Sum/1
  Abs1/1 -> Sum/2
  x/1 -> Abs/1
  y/1 -> Abs2/1
  Abs/1 -> Compare To Constant/1
  Abs2/1 -> Compare To Constant1/1
  z/1 -> Compare To Constant2/1
  Compare To Constant1/1 -> Logical Operator/2
  Compare To Constant/1 -> Logical Operator/1
  Compare To Constant2/1 -> Logical Operator/3
  Logical Operator/1 -> Display/1, Enable/1

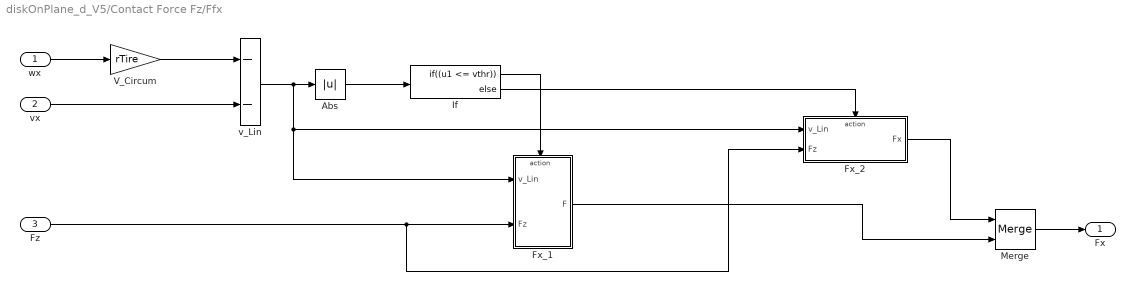
== system diskOnPlane_d_V5/Contact Force Fz/Ffx ==
  wx : Inport
  vx : Inport  Port=2
  Fz : Inport  Port=3
  Abs : Abs
  Fx_1 : Subsystem  AncestorBlock=Contact_Forces_Lib/2D/Circle to Finite Line Force/No Force
  Fx_2 : Subsystem
  If : If  IfExpression=(u1 <= vthr)
  Merge : Merge
  V_Circum : Gain  Gain=rTire
  v_Lin : Sum  Inputs=--
  Fx : Outport
  wires:
  wx/1 -> V_Circum/1
  V_Circum/1 -> v_Lin/1
  vx/1 -> v_Lin/2
  v_Lin/1 -> Fx_2/1(v_Lin), Fx_1/1(v_Lin), Abs/1
  Abs/1 -> If/1
  If/1 -> Fx_1/Action
  Fz/1 -> Fx_2/2(Fz), Fx_1/2(Fz)
  If/2 -> Fx_2/Action
  Merge/1 -> Fx/1
  Fx_1/1(F) -> Merge/2
  Fx_2/1(Fx) -> Merge/1

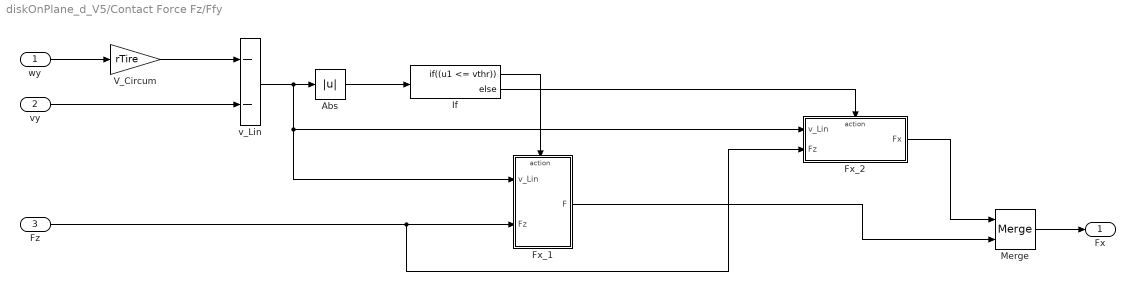
== system diskOnPlane_d_V5/Contact Force Fz/Ffy ==
  wy : Inport
  vy : Inport  Port=2
  Fz : Inport  Port=3
  Abs : Abs
  Fx_1 : Subsystem  AncestorBlock=Contact_Forces_Lib/2D/Circle to Finite Line Force/No Force
  Fx_2 : Subsystem
  If : If  IfExpression=(u1 <= vthr)
  Merge : Merge
  V_Circum : Gain  Gain=rTire
  v_Lin : Sum  Inputs=--
  Fx : Outport
  wires:
  Fx_2/1(Fx) -> Merge/1
  Fx_1/1(F) -> Merge/2
  Merge/1 -> Fx/1
  If/2 -> Fx_2/Action
  Fz/1 -> Fx_1/2(Fz), Fx_2/2(Fz)
  If/1 -> Fx_1/Action
  Abs/1 -> If/1
  v_Lin/1 -> Abs/1, Fx_1/1(v_Lin), Fx_2/1(v_Lin)
  vy/1 -> v_Lin/2
  V_Circum/1 -> v_Lin/1
  wy/1 -> V_Circum/1

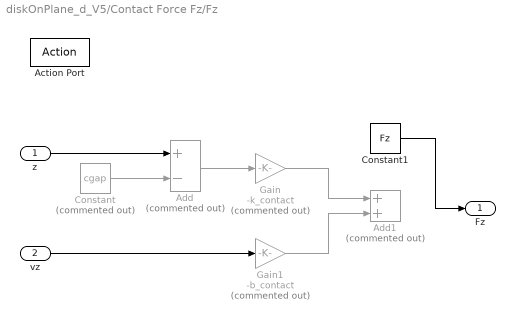
== system diskOnPlane_d_V5/Contact Force Fz/Fz ==
  z : Inport
  vz : Inport  Port=2
  Action Port : ActionPort  ActionType=then
  Add : Sum  Commented=on  Inputs=+-
  Add1 : Sum  Commented=on
  Constant : Constant  Commented=on  Value=cgap
  Constant1 : Constant  Value=Fz
  Gain : Gain  Commented=on  Gain=-k_contact
  Gain1 : Gain  Commented=on  Gain=-b_contact
  Fz : Outport
  wires:
  z/1 -> Add/1
  Constant/1 -> Add/2
  Add/1 -> Gain/1
  vz/1 -> Gain1/1
  Gain/1 -> Add1/1
  Gain1/1 -> Add1/2
  Constant1/1 -> Fz/1

== system diskOnPlane_d_V5/Contact Force Fz/No Force ==
  Action Port : ActionPort  ActionType=else
  Zeros : Constant  Value=0  SampleTime=0
  F : Outport  InitialOutput=0
  wires:
  Zeros/1 -> F/1

== system diskOnPlane_d_V5/Iniital Torque/Signal Builder ==
  Demux : Demux  Tag=STV Demux  Outputs=1
  FromWs : FromWorkspace  Tag=STV FromWs  VariableName=tuvar  SampleTime=0
      SigBuilderData=|
      | common.afterFinalStr = 'Extrapolate'
      | common.sampleTime = 0
      | dataSet.timeRange = [0 10]
      | dataSet.name = 'Group 1'
      | sbobj.Groups.Name = 'Group 1'
      | sbobj.Groups.Signals.Name = 'Signal 1'
      | sbobj.Groups.Signals.XData = [0 1 1 10]
      | sbobj.Groups.Signals.YData = [-500 -500 0 0]
  Signal 1 : Outport  Tag=STV Outport
  wires:
  Demux/1 -> Signal 1/1
  FromWs/1 -> Demux/1

== system diskOnPlane_d_V5/plane/Plane ==
  Plane : sm_lib/Body Elements/Solid  InertiaType=CalculateFromGeometry  Mass=1  MassUnits=kg  CenterOfMass=[0 0 0]  CenterOfMassUnits=m  MomentsOfInertia=[1 1 1]  MomentsOfInertiaUnits=kg*m^2  ProductsOfInertia=[0 0 0]  ProductsOfInertiaUnits=kg*m^2  DensityBased=on  Density=1000  DensityUnits=kg/(m^3)  DoExposeReferenceFrame=on  SerializedFrames=<Frames/>  GraphicType=FromGeometry  MarkerShape=Sphere  MarkerSize=10  MarkerSizeUnits=m  GraphicVisPropType=SimpleVisualProperties  GraphicDiffuseColor=[0.5 0.5 0.5]  GraphicSpecularColor=[0.5 0.5 0.5 1.0]  GraphicAmbientColor=[0.15 0.15 0.15 1.0]  GraphicEmissiveColor=[0.0 0.0 0.0 1.0]  GraphicShininess=75  GraphicOpacity=0.5  GeometryShape=Brick  RectangleSize=[1 1]  RectangleSizeUnits=m  BrickDimensions=[xPlaLgt yPlaLgt zPlaLgt]  BrickDimensionUnits=m  CylinderRadius=1  CylinderRadiusUnits=m  CylinderLength=1  CylinderLengthUnits=m  SphereRadius=1  SphereRadiusUnits=m  EllipsoidRadii=[1 1 1]  EllipsoidRadiiUnits=m  ExtrusionCrossSection=[1 1; -1 1; -1 -1; 1 -1]  ExtrusionCrossSectionUnits=m  ExtrusionLength=1  ExtrusionLengthUnits=m  PolygonNumSides=3  PolygonOuterRadius=1  PolygonOuterRadiusUnits=m  ExtGeomFileType=STL  ExtGeomFileUnits=m  RevolutionCrossSection=[1 1; 1 -1; 2 -1; 2 1]  RevolutionCrossSectionUnits=m  RevolutionExtent=Full  RevolutionAngle=180  RevolutionAngleUnits=deg
  F : PMIOPort  Port=1  Side=Right
  B : PMIOPort  Port=2  Side=Left
  connections:
  Plane/RConn1 -- F/RConn1 -- B/RConn1

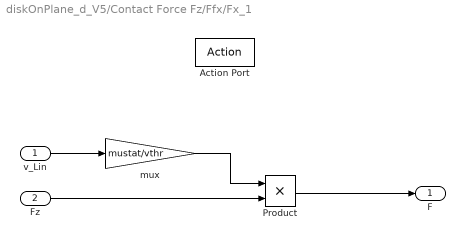
== system diskOnPlane_d_V5/Contact Force Fz/Ffx/Fx_1 ==
  v_Lin : Inport
  Fz : Inport  Port=2
  Action Port : ActionPort  ActionType=then
  Product : Product
  mux : Gain  Gain=mustat/vthr
  F : Outport  InitialOutput=0
  wires:
  v_Lin/1 -> mux/1
  Fz/1 -> Product/2
  mux/1 -> Product/1
  Product/1 -> F/1

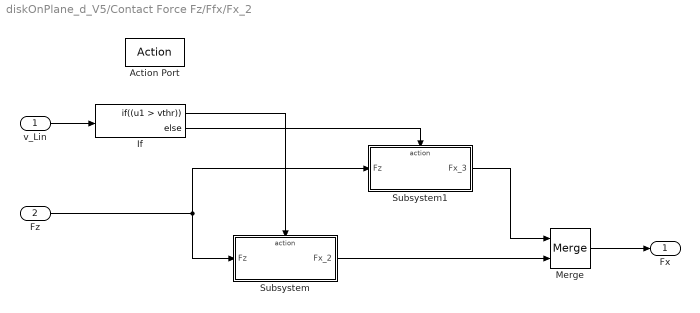
== system diskOnPlane_d_V5/Contact Force Fz/Ffx/Fx_2 ==
  v_Lin : Inport
  Fz : Inport  Port=2
  Action Port : ActionPort  ActionType=else
  If : If  IfExpression=(u1 > vthr)
  Merge : Merge
  Subsystem : Subsystem
  Subsystem1 : Subsystem
  Fx : Outport
  wires:
  v_Lin/1 -> If/1
  If/1 -> Subsystem/Action
  Fz/1 -> Subsystem1/1(Fz), Subsystem/1(Fz)
  If/2 -> Subsystem1/Action
  Subsystem/1(Fx_2) -> Merge/2
  Subsystem1/1(Fx_3) -> Merge/1
  Merge/1 -> Fx/1

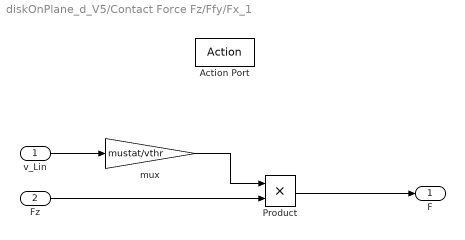
== system diskOnPlane_d_V5/Contact Force Fz/Ffy/Fx_1 ==
  v_Lin : Inport
  Fz : Inport  Port=2
  Action Port : ActionPort  ActionType=then
  Product : Product
  mux : Gain  Gain=mustat/vthr
  F : Outport  InitialOutput=0
  wires:
  Product/1 -> F/1
  mux/1 -> Product/1
  Fz/1 -> Product/2
  v_Lin/1 -> mux/1

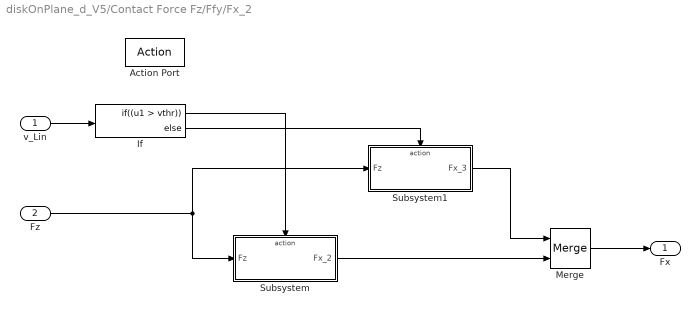
== system diskOnPlane_d_V5/Contact Force Fz/Ffy/Fx_2 ==
  v_Lin : Inport
  Fz : Inport  Port=2
  Action Port : ActionPort  ActionType=else
  If : If  IfExpression=(u1 > vthr)
  Merge : Merge
  Subsystem : Subsystem
  Subsystem1 : Subsystem
  Fx : Outport
  wires:
  Merge/1 -> Fx/1
  Subsystem1/1(Fx_3) -> Merge/1
  Subsystem/1(Fx_2) -> Merge/2
  If/2 -> Subsystem1/Action
  Fz/1 -> Subsystem/1(Fz), Subsystem1/1(Fz)
  If/1 -> Subsystem/Action
  v_Lin/1 -> If/1

== system diskOnPlane_d_V5/Contact Force Fz/Ffx/Fx_2/Subsystem ==
  Fz : Inport
  Action Port : ActionPort  ActionType=then
  Gain : Gain  Gain=mustat
  Fx_2 : Outport
  wires:
  Fz/1 -> Gain/1
  Gain/1 -> Fx_2/1

== system diskOnPlane_d_V5/Contact Force Fz/Ffx/Fx_2/Subsystem1 ==
  Fz : Inport
  Action Port : ActionPort  ActionType=else
  Gain : Gain  Gain=-mustat
  Fx_3 : Outport
  wires:
  Fz/1 -> Gain/1
  Gain/1 -> Fx_3/1

== system diskOnPlane_d_V5/Contact Force Fz/Ffy/Fx_2/Subsystem ==
  Fz : Inport
  Action Port : ActionPort  ActionType=then
  Gain : Gain  Gain=mustat
  Fx_2 : Outport
  wires:
  Gain/1 -> Fx_2/1
  Fz/1 -> Gain/1

== system diskOnPlane_d_V5/Contact Force Fz/Ffy/Fx_2/Subsystem1 ==
  Fz : Inport
  Action Port : ActionPort  ActionType=else
  Gain : Gain  Gain=-mustat
  Fx_3 : Outport
  wires:
  Gain/1 -> Fx_3/1
  Fz/1 -> Gain/1
